simulink library "Common_Library"  (Simulink 8.1)
settings: Solver=ode45  StartTime=0.0  StopTime=10.0  RelTol=1e-3
values from neighbouring files (symbols this model uses):
  address_0x00 = MOVcr    [ROM.m]
  address_0x01 = 10    [ROM.m]
  address_0x02 = REG_A    [ROM.m]
  address_0x03 = MOVcr    [ROM.m]
  address_0x04 = 3    [ROM.m]
  address_0x05 = REG_B    [ROM.m]
  address_0x06 = ADDcr    [ROM.m]
  address_0x07 = 50    [ROM.m]
  address_0x08 = REG_B    [ROM.m]
  address_0x09 = ADDrr    [ROM.m]
  address_0x0A = REG_A    [ROM.m]
  address_0x0B = REG_B    [ROM.m]
  address_0x0C = 0    [ROM.m]
  address_0x0D = 0    [ROM.m]
  address_0x0E = 0    [ROM.m]
  address_0x0F = 177    [ROM.m]
libraries: Common_Library x115, Computer_Library x85, commutil2 x67, simulink_extras x1
(part 3 of 3)

== system Common_Library/Multiplexers/2_to_1_Bit_Multiplexer ==
  Address(1b) : Inport
  Data_In_1(1b) : Inport  Port=2
  Data_In_0(1b) : Inport  Port=3
  Logical Operator12 : Logic  Operator=NOT  Inputs=4  IconShape=distinctive  AllPortsSameDT=off  OutDataTypeStr=boolean
  Logical Operator2 : Logic  IconShape=distinctive  AllPortsSameDT=off  OutDataTypeStr=boolean
  Logical Operator3 : Logic  IconShape=distinctive  AllPortsSameDT=off  OutDataTypeStr=boolean
  Logical Operator8 : Logic  Operator=OR  IconShape=distinctive  OutDataTypeStr=boolean
  Data_Out(1b) : Outport
  wires:
  Logical Operator12/1 -> Logical Operator3/2
  Address(1b)/1 -> Logical Operator2/2, Logical Operator12/1
  Logical Operator8/1 -> Data_Out(1b)/1
  Data_In_1(1b)/1 -> Logical Operator2/1
  Data_In_0(1b)/1 -> Logical Operator3/1
  Logical Operator3/1 -> Logical Operator8/2
  Logical Operator2/1 -> Logical Operator8/1

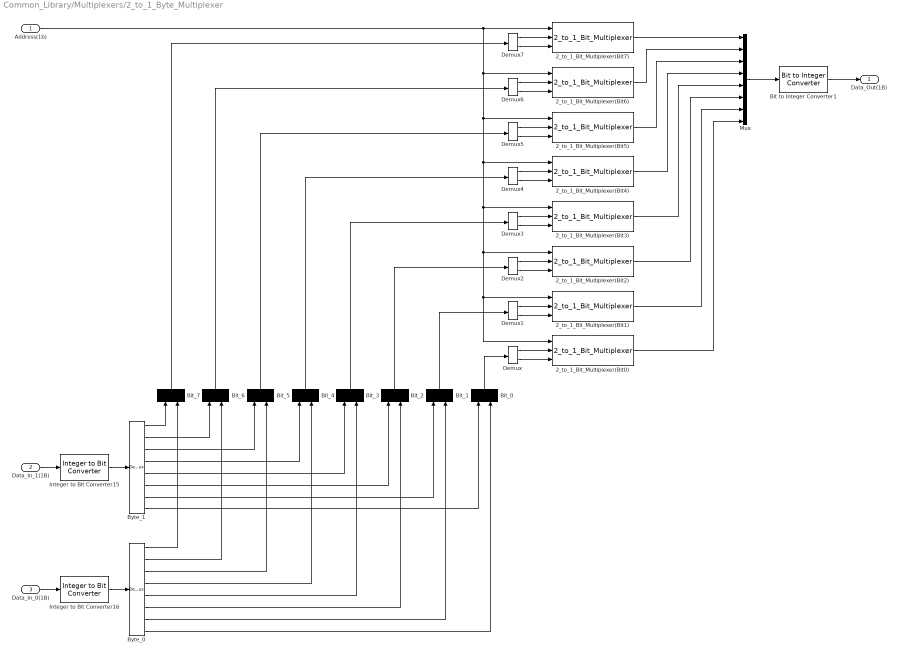
== system Common_Library/Multiplexers/2_to_1_Byte_Multiplexer ==
  Address(1b) : Inport
  Data_In_1(1B) : Inport  Port=2
  Data_In_0(1B) : Inport  Port=3
  2_to_1_Bit_Multiplexer(Bit0) : Common_Library/Multiplexers/2_to_1_Bit_Multiplexer
  2_to_1_Bit_Multiplexer(Bit1) : Common_Library/Multiplexers/2_to_1_Bit_Multiplexer
  2_to_1_Bit_Multiplexer(Bit2) : Common_Library/Multiplexers/2_to_1_Bit_Multiplexer
  2_to_1_Bit_Multiplexer(Bit3) : Common_Library/Multiplexers/2_to_1_Bit_Multiplexer
  2_to_1_Bit_Multiplexer(Bit4) : Common_Library/Multiplexers/2_to_1_Bit_Multiplexer
  2_to_1_Bit_Multiplexer(Bit5) : Common_Library/Multiplexers/2_to_1_Bit_Multiplexer
  2_to_1_Bit_Multiplexer(Bit6) : Common_Library/Multiplexers/2_to_1_Bit_Multiplexer
  2_to_1_Bit_Multiplexer(Bit7) : Common_Library/Multiplexers/2_to_1_Bit_Multiplexer
  Bit to Integer Converter1 : commutil2/Bit to Integer Converter  nbits=8  bitOrder=MSB first  signedOutputValues=Unsigned  outDtype=uint8  outDtypeSigned=Inherit via internal rule
  Bit_{0..7} (8 alike) : Mux  Inputs=2
  Byte_0 : Demux  Outputs=8
  Byte_1 : Demux  Outputs=8
  Demux{,1..7} (8 alike) : Demux  Outputs=2
  Integer to Bit Converter15 : commutil2/Integer to Bit Converter  nbits=8  signedInputValues=Unsigned  bitOrder=MSB first  outDtype=boolean
  Integer to Bit Converter16 : commutil2/Integer to Bit Converter  nbits=8  signedInputValues=Unsigned  bitOrder=MSB first  outDtype=boolean
  Mux : Mux  Inputs=8
  Data_Out(1B) : Outport
  wires:
  Mux/1 -> Bit to Integer Converter1/1
  Bit to Integer Converter1/1 -> Data_Out(1B)/1
  Bit_0/1 -> Demux/1
  Bit_1/1 -> Demux1/1
  Bit_2/1 -> Demux2/1
  Bit_3/1 -> Demux3/1
  Bit_4/1 -> Demux4/1
  Bit_5/1 -> Demux5/1
  Bit_6/1 -> Demux6/1
  Bit_7/1 -> Demux7/1
  Address(1b)/1 -> 2_to_1_Bit_Multiplexer(Bit7)/1, 2_to_1_Bit_Multiplexer(Bit0)/1, 2_to_1_Bit_Multiplexer(Bit1)/1, 2_to_1_Bit_Multiplexer(Bit2)/1, 2_to_1_Bit_Multiplexer(Bit3)/1, 2_to_1_Bit_Multiplexer(Bit4)/1, 2_to_1_Bit_Multiplexer(Bit5)/1, 2_to_1_Bit_Multiplexer(Bit6)/1
  2_to_1_Bit_Multiplexer(Bit4)/1 -> Mux/4
  2_to_1_Bit_Multiplexer(Bit5)/1 -> Mux/3
  2_to_1_Bit_Multiplexer(Bit6)/1 -> Mux/2
  2_to_1_Bit_Multiplexer(Bit7)/1 -> Mux/1
  2_to_1_Bit_Multiplexer(Bit3)/1 -> Mux/5
  2_to_1_Bit_Multiplexer(Bit2)/1 -> Mux/6
  2_to_1_Bit_Multiplexer(Bit1)/1 -> Mux/7
  2_to_1_Bit_Multiplexer(Bit0)/1 -> Mux/8
  Byte_0/8 -> Bit_0/2
  Byte_1/8 -> Bit_0/1
  Byte_0/7 -> Bit_1/2
  Byte_1/7 -> Bit_1/1
  Byte_0/6 -> Bit_2/2
  Byte_1/6 -> Bit_2/1
  Byte_0/5 -> Bit_3/2
  Byte_1/5 -> Bit_3/1
  Byte_0/4 -> Bit_4/2
  Byte_1/4 -> Bit_4/1
  Byte_0/3 -> Bit_5/2
  Byte_1/3 -> Bit_5/1
  Byte_0/2 -> Bit_6/2
  Byte_1/2 -> Bit_6/1
  Byte_0/1 -> Bit_7/2
  Byte_1/1 -> Bit_7/1
  Integer to Bit Converter15/1 -> Byte_1/1
  Data_In_1(1B)/1 -> Integer to Bit Converter15/1
  Integer to Bit Converter16/1 -> Byte_0/1
  Data_In_0(1B)/1 -> Integer to Bit Converter16/1
  Demux/1 -> 2_to_1_Bit_Multiplexer(Bit0)/2
  Demux/2 -> 2_to_1_Bit_Multiplexer(Bit0)/3
  Demux1/1 -> 2_to_1_Bit_Multiplexer(Bit1)/2
  Demux1/2 -> 2_to_1_Bit_Multiplexer(Bit1)/3
  Demux2/1 -> 2_to_1_Bit_Multiplexer(Bit2)/2
  Demux2/2 -> 2_to_1_Bit_Multiplexer(Bit2)/3
  Demux3/2 -> 2_to_1_Bit_Multiplexer(Bit3)/3
  Demux3/1 -> 2_to_1_Bit_Multiplexer(Bit3)/2
  Demux4/2 -> 2_to_1_Bit_Multiplexer(Bit4)/3
  Demux4/1 -> 2_to_1_Bit_Multiplexer(Bit4)/2
  Demux5/1 -> 2_to_1_Bit_Multiplexer(Bit5)/2
  Demux5/2 -> 2_to_1_Bit_Multiplexer(Bit5)/3
  Demux6/1 -> 2_to_1_Bit_Multiplexer(Bit6)/2
  Demux6/2 -> 2_to_1_Bit_Multiplexer(Bit6)/3
  Demux7/2 -> 2_to_1_Bit_Multiplexer(Bit7)/3
  Demux7/1 -> 2_to_1_Bit_Multiplexer(Bit7)/2

== system Common_Library/Multiplexers/4_to_1_Bit_Multiplexer ==
  Address_1(1b) : Inport
  Address_0(1b) : Inport  Port=2
  Data_In_3(1b) : Inport  Port=3
  Data_In_2(1b) : Inport  Port=4
  Data_In_1(1b) : Inport  Port=5
  Data_In_0(1b) : Inport  Port=6
  Logical Operator{,1..3} (4 alike) : Logic  Inputs=3  IconShape=distinctive  AllPortsSameDT=off  OutDataTypeStr=boolean
  Logical Operator11 : Logic  Operator=NOT  Inputs=4  IconShape=distinctive  AllPortsSameDT=off  OutDataTypeStr=boolean
  Logical Operator12 : Logic  Operator=NOT  Inputs=4  IconShape=distinctive  AllPortsSameDT=off  OutDataTypeStr=boolean
  Logical Operator8 : Logic  Operator=OR  Inputs=4  IconShape=distinctive  OutDataTypeStr=boolean
  Data_Out(1b) : Outport
  wires:
  Logical Operator12/1 -> Logical Operator3/2, Logical Operator1/2
  Address_0(1b)/1 -> Logical Operator/2, Logical Operator2/2, Logical Operator12/1
  Logical Operator11/1 -> Logical Operator3/3, Logical Operator2/3
  Address_1(1b)/1 -> Logical Operator/3, Logical Operator1/3, Logical Operator11/1
  Logical Operator8/1 -> Data_Out(1b)/1
  Data_In_3(1b)/1 -> Logical Operator/1
  Data_In_2(1b)/1 -> Logical Operator1/1
  Data_In_1(1b)/1 -> Logical Operator2/1
  Data_In_0(1b)/1 -> Logical Operator3/1
  Logical Operator3/1 -> Logical Operator8/4
  Logical Operator2/1 -> Logical Operator8/3
  Logical Operator1/1 -> Logical Operator8/2
  Logical Operator/1 -> Logical Operator8/1

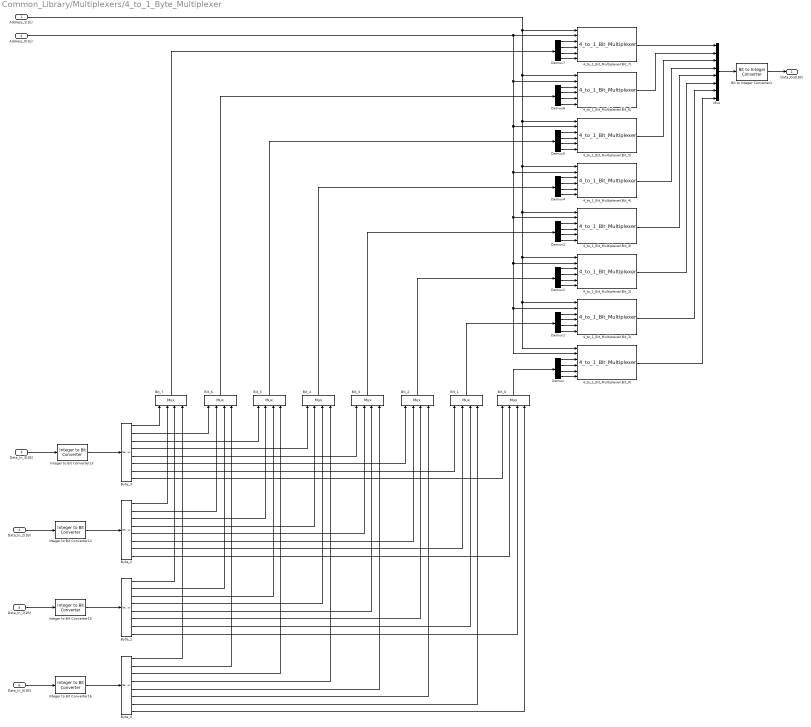
== system Common_Library/Multiplexers/4_to_1_Byte_Multiplexer ==
  Address_1(1b) : Inport
  Address_0(1b) : Inport  Port=2
  Data_In_3(1B) : Inport  Port=3
  Data_In_2(1B) : Inport  Port=4
  Data_In_1(1B) : Inport  Port=5
  Data_In_0(1B) : Inport  Port=6
  4_to_1_Bit_Multiplexer(Bit_0) : Common_Library/Multiplexers/4_to_1_Bit_Multiplexer
  4_to_1_Bit_Multiplexer(Bit_1) : Common_Library/Multiplexers/4_to_1_Bit_Multiplexer
  4_to_1_Bit_Multiplexer(Bit_2) : Common_Library/Multiplexers/4_to_1_Bit_Multiplexer
  4_to_1_Bit_Multiplexer(Bit_3) : Common_Library/Multiplexers/4_to_1_Bit_Multiplexer
  4_to_1_Bit_Multiplexer(Bit_4) : Common_Library/Multiplexers/4_to_1_Bit_Multiplexer
  4_to_1_Bit_Multiplexer(Bit_5) : Common_Library/Multiplexers/4_to_1_Bit_Multiplexer
  4_to_1_Bit_Multiplexer(Bit_6) : Common_Library/Multiplexers/4_to_1_Bit_Multiplexer
  4_to_1_Bit_Multiplexer(Bit_7) : Common_Library/Multiplexers/4_to_1_Bit_Multiplexer
  Bit to Integer Converter1 : commutil2/Bit to Integer Converter  nbits=8  bitOrder=MSB first  signedOutputValues=Unsigned  outDtype=uint8  outDtypeSigned=Inherit via internal rule
  Bit_{0..7} (8 alike) : Mux
  Byte_{0..3} (4 alike) : Demux  Outputs=8
  Demux{,1..7} (8 alike) : Demux
  Integer to Bit Converter{13..16} (4 alike) : commutil2/Integer to Bit Converter  nbits=8  signedInputValues=Unsigned  bitOrder=MSB first  outDtype=boolean
  Mux : Mux  Inputs=8
  Data_Out(1B) : Outport
  wires:
  Mux/1 -> Bit to Integer Converter1/1
  Bit to Integer Converter1/1 -> Data_Out(1B)/1
  Bit_0/1 -> Demux/1
  Bit_1/1 -> Demux1/1
  Bit_2/1 -> Demux2/1
  Bit_3/1 -> Demux3/1
  Bit_4/1 -> Demux4/1
  Bit_5/1 -> Demux5/1
  Bit_6/1 -> Demux6/1
  Bit_7/1 -> Demux7/1
  Address_0(1b)/1 -> 4_to_1_Bit_Multiplexer(Bit_7)/2, 4_to_1_Bit_Multiplexer(Bit_0)/2, 4_to_1_Bit_Multiplexer(Bit_1)/2, 4_to_1_Bit_Multiplexer(Bit_2)/2, 4_to_1_Bit_Multiplexer(Bit_3)/2, 4_to_1_Bit_Multiplexer(Bit_4)/2, 4_to_1_Bit_Multiplexer(Bit_5)/2, 4_to_1_Bit_Multiplexer(Bit_6)/2
  Address_1(1b)/1 -> 4_to_1_Bit_Multiplexer(Bit_7)/1, 4_to_1_Bit_Multiplexer(Bit_0)/1, 4_to_1_Bit_Multiplexer(Bit_1)/1, 4_to_1_Bit_Multiplexer(Bit_2)/1, 4_to_1_Bit_Multiplexer(Bit_3)/1, 4_to_1_Bit_Multiplexer(Bit_4)/1, 4_to_1_Bit_Multiplexer(Bit_5)/1, 4_to_1_Bit_Multiplexer(Bit_6)/1
  4_to_1_Bit_Multiplexer(Bit_4)/1 -> Mux/4
  4_to_1_Bit_Multiplexer(Bit_5)/1 -> Mux/3
  4_to_1_Bit_Multiplexer(Bit_6)/1 -> Mux/2
  4_to_1_Bit_Multiplexer(Bit_7)/1 -> Mux/1
  4_to_1_Bit_Multiplexer(Bit_3)/1 -> Mux/5
  4_to_1_Bit_Multiplexer(Bit_2)/1 -> Mux/6
  4_to_1_Bit_Multiplexer(Bit_1)/1 -> Mux/7
  4_to_1_Bit_Multiplexer(Bit_0)/1 -> Mux/8
  Byte_0/8 -> Bit_0/4
  Byte_1/8 -> Bit_0/3
  Byte_2/8 -> Bit_0/2
  Byte_3/8 -> Bit_0/1
  Byte_0/7 -> Bit_1/4
  Byte_1/7 -> Bit_1/3
  Byte_2/7 -> Bit_1/2
  Byte_3/7 -> Bit_1/1
  Byte_0/6 -> Bit_2/4
  Byte_1/6 -> Bit_2/3
  Byte_2/6 -> Bit_2/2
  Byte_3/6 -> Bit_2/1
  Byte_0/5 -> Bit_3/4
  Byte_1/5 -> Bit_3/3
  Byte_2/5 -> Bit_3/2
  Byte_3/5 -> Bit_3/1
  Byte_0/4 -> Bit_4/4
  Byte_1/4 -> Bit_4/3
  Byte_2/4 -> Bit_4/2
  Byte_3/4 -> Bit_4/1
  Byte_0/3 -> Bit_5/4
  Byte_1/3 -> Bit_5/3
  Byte_2/3 -> Bit_5/2
  Byte_3/3 -> Bit_5/1
  Byte_0/2 -> Bit_6/4
  Byte_1/2 -> Bit_6/3
  Byte_2/2 -> Bit_6/2
  Byte_3/2 -> Bit_6/1
  Byte_0/1 -> Bit_7/4
  Byte_1/1 -> Bit_7/3
  Byte_2/1 -> Bit_7/2
  Byte_3/1 -> Bit_7/1
  Integer to Bit Converter13/1 -> Byte_3/1
  Data_In_3(1B)/1 -> Integer to Bit Converter13/1
  Integer to Bit Converter14/1 -> Byte_2/1
  Data_In_2(1B)/1 -> Integer to Bit Converter14/1
  Integer to Bit Converter15/1 -> Byte_1/1
  Data_In_1(1B)/1 -> Integer to Bit Converter15/1
  Integer to Bit Converter16/1 -> Byte_0/1
  Data_In_0(1B)/1 -> Integer to Bit Converter16/1
  Demux/1 -> 4_to_1_Bit_Multiplexer(Bit_0)/3
  Demux/2 -> 4_to_1_Bit_Multiplexer(Bit_0)/4
  Demux/3 -> 4_to_1_Bit_Multiplexer(Bit_0)/5
  Demux/4 -> 4_to_1_Bit_Multiplexer(Bit_0)/6
  Demux1/1 -> 4_to_1_Bit_Multiplexer(Bit_1)/3
  Demux1/2 -> 4_to_1_Bit_Multiplexer(Bit_1)/4
  Demux1/3 -> 4_to_1_Bit_Multiplexer(Bit_1)/5
  Demux1/4 -> 4_to_1_Bit_Multiplexer(Bit_1)/6
  Demux2/1 -> 4_to_1_Bit_Multiplexer(Bit_2)/3
  Demux2/2 -> 4_to_1_Bit_Multiplexer(Bit_2)/4
  Demux2/3 -> 4_to_1_Bit_Multiplexer(Bit_2)/5
  Demux2/4 -> 4_to_1_Bit_Multiplexer(Bit_2)/6
  Demux3/1 -> 4_to_1_Bit_Multiplexer(Bit_3)/3
  Demux3/2 -> 4_to_1_Bit_Multiplexer(Bit_3)/4
  Demux3/3 -> 4_to_1_Bit_Multiplexer(Bit_3)/5
  Demux3/4 -> 4_to_1_Bit_Multiplexer(Bit_3)/6
  Demux4/1 -> 4_to_1_Bit_Multiplexer(Bit_4)/3
  Demux4/2 -> 4_to_1_Bit_Multiplexer(Bit_4)/4
  Demux4/3 -> 4_to_1_Bit_Multiplexer(Bit_4)/5
  Demux4/4 -> 4_to_1_Bit_Multiplexer(Bit_4)/6
  Demux5/1 -> 4_to_1_Bit_Multiplexer(Bit_5)/3
  Demux5/2 -> 4_to_1_Bit_Multiplexer(Bit_5)/4
  Demux5/3 -> 4_to_1_Bit_Multiplexer(Bit_5)/5
  Demux5/4 -> 4_to_1_Bit_Multiplexer(Bit_5)/6
  Demux6/1 -> 4_to_1_Bit_Multiplexer(Bit_6)/3
  Demux6/2 -> 4_to_1_Bit_Multiplexer(Bit_6)/4
  Demux6/3 -> 4_to_1_Bit_Multiplexer(Bit_6)/5
  Demux6/4 -> 4_to_1_Bit_Multiplexer(Bit_6)/6
  Demux7/1 -> 4_to_1_Bit_Multiplexer(Bit_7)/3
  Demux7/2 -> 4_to_1_Bit_Multiplexer(Bit_7)/4
  Demux7/3 -> 4_to_1_Bit_Multiplexer(Bit_7)/5
  Demux7/4 -> 4_to_1_Bit_Multiplexer(Bit_7)/6

== system Common_Library/Multiplexers/8_to_1_Bit_Multiplexer ==
  Address_2(1b) : Inport
  Address_1(1b) : Inport  Port=2
  Address_0(1b) : Inport  Port=3
  Data_In_7(1b) : Inport  Port=4
  Data_In_6(1b) : Inport  Port=5
  Data_In_5(1b) : Inport  Port=6
  Data_In_4(1b) : Inport  Port=7
  Data_In_3(1b) : Inport  Port=8
  Data_In_2(1b) : Inport  Port=9
  Data_In_1(1b) : Inport  Port=10
  Data_In_0(1b) : Inport  Port=11
  Logical Operator{,1..7} (8 alike) : Logic  Inputs=4  IconShape=distinctive  AllPortsSameDT=off  OutDataTypeStr=boolean
  Logical Operator10 : Logic  Operator=NOT  Inputs=4  IconShape=distinctive  AllPortsSameDT=off  OutDataTypeStr=boolean
  Logical Operator11 : Logic  Operator=NOT  Inputs=4  IconShape=distinctive  AllPortsSameDT=off  OutDataTypeStr=boolean
  Logical Operator12 : Logic  Operator=NOT  Inputs=4  IconShape=distinctive  AllPortsSameDT=off  OutDataTypeStr=boolean
  Logical Operator8 : Logic  Operator=OR  Inputs=8  IconShape=distinctive  OutDataTypeStr=boolean
  Data_Out(1b) : Outport
  wires:
  Logical Operator12/1 -> Logical Operator1/2, Logical Operator3/2, Logical Operator5/2, Logical Operator7/2
  Address_0(1b)/1 -> Logical Operator/2, Logical Operator2/2, Logical Operator4/2, Logical Operator6/2, Logical Operator12/1
  Logical Operator11/1 -> Logical Operator2/4, Logical Operator3/4, Logical Operator6/4, Logical Operator7/4
  Address_1(1b)/1 -> Logical Operator1/4, Logical Operator4/4, Logical Operator5/4, Logical Operator/4, Logical Operator11/1
  Logical Operator10/1 -> Logical Operator4/3, Logical Operator5/3, Logical Operator6/3, Logical Operator7/3
  Address_2(1b)/1 -> Logical Operator3/3, Logical Operator2/3, Logical Operator1/3, Logical Operator/3, Logical Operator10/1
  Logical Operator8/1 -> Data_Out(1b)/1
  Data_In_7(1b)/1 -> Logical Operator/1
  Data_In_6(1b)/1 -> Logical Operator1/1
  Data_In_5(1b)/1 -> Logical Operator2/1
  Data_In_4(1b)/1 -> Logical Operator3/1
  Data_In_3(1b)/1 -> Logical Operator4/1
  Data_In_2(1b)/1 -> Logical Operator5/1
  Data_In_1(1b)/1 -> Logical Operator6/1
  Data_In_0(1b)/1 -> Logical Operator7/1
  Logical Operator7/1 -> Logical Operator8/8
  Logical Operator6/1 -> Logical Operator8/7
  Logical Operator5/1 -> Logical Operator8/6
  Logical Operator4/1 -> Logical Operator8/5
  Logical Operator3/1 -> Logical Operator8/4
  Logical Operator2/1 -> Logical Operator8/3
  Logical Operator1/1 -> Logical Operator8/2
  Logical Operator/1 -> Logical Operator8/1

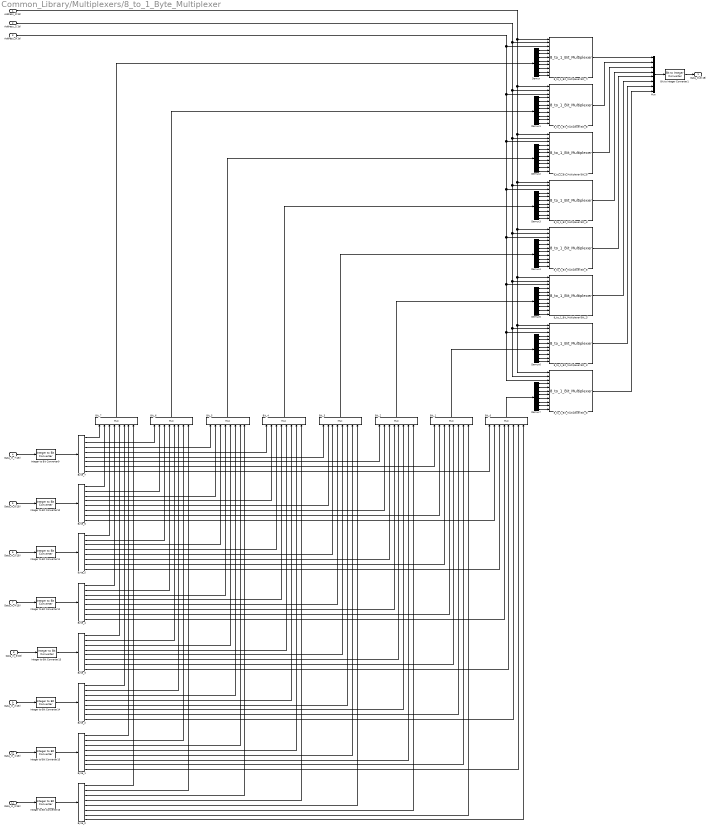
== system Common_Library/Multiplexers/8_to_1_Byte_Multiplexer ==
  Address_2(1b) : Inport
  Address_1(1b) : Inport  Port=2
  Address_0(1b) : Inport  Port=3
  Data_In_7(1B) : Inport  Port=4
  Data_In_6(1B) : Inport  Port=5
  Data_In_5(1B) : Inport  Port=6
  Data_In_4(1B) : Inport  Port=7
  Data_In_3(1B) : Inport  Port=8
  Data_In_2(1B) : Inport  Port=9
  Data_In_1(1B) : Inport  Port=10
  Data_In_0(1B) : Inport  Port=11
  8_to_1_Bit_Multiplexer(Bit_0) : Common_Library/Multiplexers/8_to_1_Bit_Multiplexer
  8_to_1_Bit_Multiplexer(Bit_1) : Common_Library/Multiplexers/8_to_1_Bit_Multiplexer
  8_to_1_Bit_Multiplexer(Bit_2) : Common_Library/Multiplexers/8_to_1_Bit_Multiplexer
  8_to_1_Bit_Multiplexer(Bit_3) : Common_Library/Multiplexers/8_to_1_Bit_Multiplexer
  8_to_1_Bit_Multiplexer(Bit_4) : Common_Library/Multiplexers/8_to_1_Bit_Multiplexer
  8_to_1_Bit_Multiplexer(Bit_5) : Common_Library/Multiplexers/8_to_1_Bit_Multiplexer
  8_to_1_Bit_Multiplexer(Bit_6) : Common_Library/Multiplexers/8_to_1_Bit_Multiplexer
  8_to_1_Bit_Multiplexer(Bit_7) : Common_Library/Multiplexers/8_to_1_Bit_Multiplexer
  Bit to Integer Converter1 : commutil2/Bit to Integer Converter  nbits=8  bitOrder=MSB first  signedOutputValues=Unsigned  outDtype=uint8  outDtypeSigned=Inherit via internal rule
  Bit_{0..7} (8 alike) : Mux  Inputs=8
  Byte_{0..7} (8 alike) : Demux  Outputs=8
  Demux{,1..7} (8 alike) : Demux  Outputs=8
  Integer to Bit Converter{9..16} (8 alike) : commutil2/Integer to Bit Converter  nbits=8  signedInputValues=Unsigned  bitOrder=MSB first  outDtype=boolean
  Mux : Mux  Inputs=8
  Data_Out(1B) : Outport
  wires:
  Mux/1 -> Bit to Integer Converter1/1
  Bit to Integer Converter1/1 -> Data_Out(1B)/1
  Bit_0/1 -> Demux7/1
  Bit_1/1 -> Demux6/1
  Bit_2/1 -> Demux5/1
  Bit_3/1 -> Demux4/1
  Bit_4/1 -> Demux3/1
  Bit_5/1 -> Demux2/1
  Bit_6/1 -> Demux1/1
  Bit_7/1 -> Demux/1
  Byte_7/7 -> Bit_1/1
  Address_0(1b)/1 -> 8_to_1_Bit_Multiplexer(Bit_0)/3, 8_to_1_Bit_Multiplexer(Bit_1)/3, 8_to_1_Bit_Multiplexer(Bit_2)/3, 8_to_1_Bit_Multiplexer(Bit_3)/3, 8_to_1_Bit_Multiplexer(Bit_4)/3, 8_to_1_Bit_Multiplexer(Bit_5)/3, 8_to_1_Bit_Multiplexer(Bit_6)/3, 8_to_1_Bit_Multiplexer(Bit_7)/3
  Address_1(1b)/1 -> 8_to_1_Bit_Multiplexer(Bit_5)/2, 8_to_1_Bit_Multiplexer(Bit_0)/2, 8_to_1_Bit_Multiplexer(Bit_1)/2, 8_to_1_Bit_Multiplexer(Bit_2)/2, 8_to_1_Bit_Multiplexer(Bit_3)/2, 8_to_1_Bit_Multiplexer(Bit_4)/2, 8_to_1_Bit_Multiplexer(Bit_6)/2, 8_to_1_Bit_Multiplexer(Bit_7)/2
  Address_2(1b)/1 -> 8_to_1_Bit_Multiplexer(Bit_0)/1, 8_to_1_Bit_Multiplexer(Bit_1)/1, 8_to_1_Bit_Multiplexer(Bit_2)/1, 8_to_1_Bit_Multiplexer(Bit_3)/1, 8_to_1_Bit_Multiplexer(Bit_4)/1, 8_to_1_Bit_Multiplexer(Bit_5)/1, 8_to_1_Bit_Multiplexer(Bit_6)/1, 8_to_1_Bit_Multiplexer(Bit_7)/1
  8_to_1_Bit_Multiplexer(Bit_4)/1 -> Mux/4
  8_to_1_Bit_Multiplexer(Bit_5)/1 -> Mux/3
  8_to_1_Bit_Multiplexer(Bit_6)/1 -> Mux/2
  8_to_1_Bit_Multiplexer(Bit_7)/1 -> Mux/1
  8_to_1_Bit_Multiplexer(Bit_3)/1 -> Mux/5
  8_to_1_Bit_Multiplexer(Bit_2)/1 -> Mux/6
  8_to_1_Bit_Multiplexer(Bit_1)/1 -> Mux/7
  8_to_1_Bit_Multiplexer(Bit_0)/1 -> Mux/8
  Byte_0/8 -> Bit_0/8
  Byte_1/8 -> Bit_0/7
  Byte_2/8 -> Bit_0/6
  Byte_3/8 -> Bit_0/5
  Byte_4/8 -> Bit_0/4
  Byte_5/8 -> Bit_0/3
  Byte_6/8 -> Bit_0/2
  Byte_7/8 -> Bit_0/1
  Byte_0/7 -> Bit_1/8
  Byte_1/7 -> Bit_1/7
  Byte_2/7 -> Bit_1/6
  Byte_3/7 -> Bit_1/5
  Byte_4/7 -> Bit_1/4
  Byte_5/7 -> Bit_1/3
  Byte_6/7 -> Bit_1/2
  Byte_0/6 -> Bit_2/8
  Byte_1/6 -> Bit_2/7
  Byte_2/6 -> Bit_2/6
  Byte_3/6 -> Bit_2/5
  Byte_4/6 -> Bit_2/4
  Byte_5/6 -> Bit_2/3
  Byte_6/6 -> Bit_2/2
  Byte_7/6 -> Bit_2/1
  Byte_0/5 -> Bit_3/8
  Byte_1/5 -> Bit_3/7
  Byte_2/5 -> Bit_3/6
  Byte_3/5 -> Bit_3/5
  Byte_4/5 -> Bit_3/4
  Byte_5/5 -> Bit_3/3
  Byte_6/5 -> Bit_3/2
  Byte_7/5 -> Bit_3/1
  Byte_0/4 -> Bit_4/8
  Byte_1/4 -> Bit_4/7
  Byte_2/4 -> Bit_4/6
  Byte_3/4 -> Bit_4/5
  Byte_4/4 -> Bit_4/4
  Byte_5/4 -> Bit_4/3
  Byte_6/4 -> Bit_4/2
  Byte_7/4 -> Bit_4/1
  Byte_0/3 -> Bit_5/8
  Byte_1/3 -> Bit_5/7
  Byte_2/3 -> Bit_5/6
  Byte_3/3 -> Bit_5/5
  Byte_4/3 -> Bit_5/4
  Byte_5/3 -> Bit_5/3
  Byte_6/3 -> Bit_5/2
  Byte_7/3 -> Bit_5/1
  Byte_0/2 -> Bit_6/8
  Byte_1/2 -> Bit_6/7
  Byte_2/2 -> Bit_6/6
  Byte_3/2 -> Bit_6/5
  Byte_4/2 -> Bit_6/4
  Byte_5/2 -> Bit_6/3
  Byte_6/2 -> Bit_6/2
  Byte_7/2 -> Bit_6/1
  Byte_0/1 -> Bit_7/8
  Byte_1/1 -> Bit_7/7
  Byte_2/1 -> Bit_7/6
  Byte_3/1 -> Bit_7/5
  Byte_4/1 -> Bit_7/4
  Byte_5/1 -> Bit_7/3
  Byte_6/1 -> Bit_7/2
  Byte_7/1 -> Bit_7/1
  Integer to Bit Converter9/1 -> Byte_7/1
  Data_In_7(1B)/1 -> Integer to Bit Converter9/1
  Integer to Bit Converter10/1 -> Byte_6/1
  Data_In_6(1B)/1 -> Integer to Bit Converter10/1
  Integer to Bit Converter11/1 -> Byte_5/1
  Data_In_5(1B)/1 -> Integer to Bit Converter11/1
  Integer to Bit Converter12/1 -> Byte_4/1
  Data_In_4(1B)/1 -> Integer to Bit Converter12/1
  Integer to Bit Converter13/1 -> Byte_3/1
  Data_In_3(1B)/1 -> Integer to Bit Converter13/1
  Integer to Bit Converter14/1 -> Byte_2/1
  Data_In_2(1B)/1 -> Integer to Bit Converter14/1
  Integer to Bit Converter15/1 -> Byte_1/1
  Data_In_1(1B)/1 -> Integer to Bit Converter15/1
  Integer to Bit Converter16/1 -> Byte_0/1
  Data_In_0(1B)/1 -> Integer to Bit Converter16/1
  Demux/1 -> 8_to_1_Bit_Multiplexer(Bit_7)/4
  Demux/2 -> 8_to_1_Bit_Multiplexer(Bit_7)/5
  Demux/3 -> 8_to_1_Bit_Multiplexer(Bit_7)/6
  Demux/4 -> 8_to_1_Bit_Multiplexer(Bit_7)/7
  Demux/5 -> 8_to_1_Bit_Multiplexer(Bit_7)/8
  Demux/6 -> 8_to_1_Bit_Multiplexer(Bit_7)/9
  Demux/7 -> 8_to_1_Bit_Multiplexer(Bit_7)/10
  Demux/8 -> 8_to_1_Bit_Multiplexer(Bit_7)/11
  Demux1/1 -> 8_to_1_Bit_Multiplexer(Bit_6)/4
  Demux1/2 -> 8_to_1_Bit_Multiplexer(Bit_6)/5
  Demux1/3 -> 8_to_1_Bit_Multiplexer(Bit_6)/6
  Demux1/4 -> 8_to_1_Bit_Multiplexer(Bit_6)/7
  Demux1/5 -> 8_to_1_Bit_Multiplexer(Bit_6)/8
  Demux1/6 -> 8_to_1_Bit_Multiplexer(Bit_6)/9
  Demux1/7 -> 8_to_1_Bit_Multiplexer(Bit_6)/10
  Demux1/8 -> 8_to_1_Bit_Multiplexer(Bit_6)/11
  Demux2/1 -> 8_to_1_Bit_Multiplexer(Bit_5)/4
  Demux2/2 -> 8_to_1_Bit_Multiplexer(Bit_5)/5
  Demux2/3 -> 8_to_1_Bit_Multiplexer(Bit_5)/6
  Demux2/4 -> 8_to_1_Bit_Multiplexer(Bit_5)/7
  Demux2/5 -> 8_to_1_Bit_Multiplexer(Bit_5)/8
  Demux2/6 -> 8_to_1_Bit_Multiplexer(Bit_5)/9
  Demux2/7 -> 8_to_1_Bit_Multiplexer(Bit_5)/10
  Demux2/8 -> 8_to_1_Bit_Multiplexer(Bit_5)/11
  Demux3/1 -> 8_to_1_Bit_Multiplexer(Bit_4)/4
  Demux3/2 -> 8_to_1_Bit_Multiplexer(Bit_4)/5
  Demux3/3 -> 8_to_1_Bit_Multiplexer(Bit_4)/6
  Demux3/4 -> 8_to_1_Bit_Multiplexer(Bit_4)/7
  Demux3/5 -> 8_to_1_Bit_Multiplexer(Bit_4)/8
  Demux3/6 -> 8_to_1_Bit_Multiplexer(Bit_4)/9
  Demux3/7 -> 8_to_1_Bit_Multiplexer(Bit_4)/10
  Demux3/8 -> 8_to_1_Bit_Multiplexer(Bit_4)/11
  Demux4/1 -> 8_to_1_Bit_Multiplexer(Bit_3)/4
  Demux4/2 -> 8_to_1_Bit_Multiplexer(Bit_3)/5
  Demux4/3 -> 8_to_1_Bit_Multiplexer(Bit_3)/6
  Demux4/4 -> 8_to_1_Bit_Multiplexer(Bit_3)/7
  Demux4/5 -> 8_to_1_Bit_Multiplexer(Bit_3)/8
  Demux4/6 -> 8_to_1_Bit_Multiplexer(Bit_3)/9
  Demux4/7 -> 8_to_1_Bit_Multiplexer(Bit_3)/10
  Demux4/8 -> 8_to_1_Bit_Multiplexer(Bit_3)/11
  Demux5/1 -> 8_to_1_Bit_Multiplexer(Bit_2)/4
  Demux5/2 -> 8_to_1_Bit_Multiplexer(Bit_2)/5
  Demux5/3 -> 8_to_1_Bit_Multiplexer(Bit_2)/6
  Demux5/4 -> 8_to_1_Bit_Multiplexer(Bit_2)/7
  Demux5/5 -> 8_to_1_Bit_Multiplexer(Bit_2)/8
  Demux5/6 -> 8_to_1_Bit_Multiplexer(Bit_2)/9
  Demux5/7 -> 8_to_1_Bit_Multiplexer(Bit_2)/10
  Demux5/8 -> 8_to_1_Bit_Multiplexer(Bit_2)/11
  Demux6/1 -> 8_to_1_Bit_Multiplexer(Bit_1)/4
  Demux6/2 -> 8_to_1_Bit_Multiplexer(Bit_1)/5
  Demux6/3 -> 8_to_1_Bit_Multiplexer(Bit_1)/6
  Demux6/4 -> 8_to_1_Bit_Multiplexer(Bit_1)/7
  Demux6/5 -> 8_to_1_Bit_Multiplexer(Bit_1)/8
  Demux6/6 -> 8_to_1_Bit_Multiplexer(Bit_1)/9
  Demux6/7 -> 8_to_1_Bit_Multiplexer(Bit_1)/10
  Demux6/8 -> 8_to_1_Bit_Multiplexer(Bit_1)/11
  Demux7/1 -> 8_to_1_Bit_Multiplexer(Bit_0)/4
  Demux7/2 -> 8_to_1_Bit_Multiplexer(Bit_0)/5
  Demux7/3 -> 8_to_1_Bit_Multiplexer(Bit_0)/6
  Demux7/4 -> 8_to_1_Bit_Multiplexer(Bit_0)/7
  Demux7/5 -> 8_to_1_Bit_Multiplexer(Bit_0)/8
  Demux7/6 -> 8_to_1_Bit_Multiplexer(Bit_0)/9
  Demux7/7 -> 8_to_1_Bit_Multiplexer(Bit_0)/10
  Demux7/8 -> 8_to_1_Bit_Multiplexer(Bit_0)/11

== system Common_Library/Multiplexers/__256_to_1_Bit_Multiplexer__ ==
  Address(8b) : Inport
  Data_In(256b) : Inport  Port=2
  16_to_1_Bit_Multiplexer{0..16} (17 alike) : Computer_Library/Multiplexers/16_to_1_Bit_Multiplexer
  Demux16 : Demux  Outputs=16
  Demux17 : Demux  Outputs=8
  Mux : Mux  Inputs=16
  Data_Out(1b) : Outport
  wires:
  Mux/1 -> 16_to_1_Bit_Multiplexer16/5
  Demux16/1 -> 16_to_1_Bit_Multiplexer0/5
  Demux16/2 -> 16_to_1_Bit_Multiplexer1/5
  Demux16/3 -> 16_to_1_Bit_Multiplexer2/5
  Demux16/4 -> 16_to_1_Bit_Multiplexer3/5
  Demux16/5 -> 16_to_1_Bit_Multiplexer4/5
  Demux16/6 -> 16_to_1_Bit_Multiplexer5/5
  Demux16/16 -> 16_to_1_Bit_Multiplexer15/5
  Demux16/15 -> 16_to_1_Bit_Multiplexer14/5
  Demux16/14 -> 16_to_1_Bit_Multiplexer13/5
  Demux16/13 -> 16_to_1_Bit_Multiplexer12/5
  Demux16/12 -> 16_to_1_Bit_Multiplexer11/5
  Demux16/11 -> 16_to_1_Bit_Multiplexer10/5
  Demux16/10 -> 16_to_1_Bit_Multiplexer9/5
  Demux16/9 -> 16_to_1_Bit_Multiplexer8/5
  Demux16/8 -> 16_to_1_Bit_Multiplexer7/5
  Demux16/7 -> 16_to_1_Bit_Multiplexer6/5
  16_to_1_Bit_Multiplexer0/1 -> Mux/1
  16_to_1_Bit_Multiplexer1/1 -> Mux/2
  16_to_1_Bit_Multiplexer2/1 -> Mux/3
  16_to_1_Bit_Multiplexer3/1 -> Mux/4
  16_to_1_Bit_Multiplexer15/1 -> Mux/16
  16_to_1_Bit_Multiplexer14/1 -> Mux/15
  16_to_1_Bit_Multiplexer13/1 -> Mux/14
  16_to_1_Bit_Multiplexer12/1 -> Mux/13
  16_to_1_Bit_Multiplexer11/1 -> Mux/12
  16_to_1_Bit_Multiplexer10/1 -> Mux/11
  16_to_1_Bit_Multiplexer9/1 -> Mux/10
  16_to_1_Bit_Multiplexer8/1 -> Mux/9
  16_to_1_Bit_Multiplexer7/1 -> Mux/8
  16_to_1_Bit_Multiplexer6/1 -> Mux/7
  16_to_1_Bit_Multiplexer5/1 -> Mux/6
  16_to_1_Bit_Multiplexer4/1 -> Mux/5
  Demux17/5 -> 16_to_1_Bit_Multiplexer0/1, 16_to_1_Bit_Multiplexer1/1, 16_to_1_Bit_Multiplexer2/1, 16_to_1_Bit_Multiplexer3/1, 16_to_1_Bit_Multiplexer4/1, 16_to_1_Bit_Multiplexer5/1, 16_to_1_Bit_Multiplexer6/1, 16_to_1_Bit_Multiplexer7/1, 16_to_1_Bit_Multiplexer8/1, 16_to_1_Bit_Multiplexer9/1, 16_to_1_Bit_Multiplexer10/1, 16_to_1_Bit_Multiplexer11/1, 16_to_1_Bit_Multiplexer12/1, 16_to_1_Bit_Multiplexer13/1, 16_to_1_Bit_Multiplexer14/1, 16_to_1_Bit_Multiplexer15/1
  Demux17/6 -> 16_to_1_Bit_Multiplexer1/2, 16_to_1_Bit_Multiplexer2/2, 16_to_1_Bit_Multiplexer3/2, 16_to_1_Bit_Multiplexer4/2, 16_to_1_Bit_Multiplexer5/2, 16_to_1_Bit_Multiplexer6/2, 16_to_1_Bit_Multiplexer7/2, 16_to_1_Bit_Multiplexer8/2, 16_to_1_Bit_Multiplexer9/2, 16_to_1_Bit_Multiplexer10/2, 16_to_1_Bit_Multiplexer11/2, 16_to_1_Bit_Multiplexer12/2, 16_to_1_Bit_Multiplexer13/2, 16_to_1_Bit_Multiplexer14/2, 16_to_1_Bit_Multiplexer15/2, 16_to_1_Bit_Multiplexer0/2
  Demux17/7 -> 16_to_1_Bit_Multiplexer0/3, 16_to_1_Bit_Multiplexer1/3, 16_to_1_Bit_Multiplexer2/3, 16_to_1_Bit_Multiplexer3/3, 16_to_1_Bit_Multiplexer4/3, 16_to_1_Bit_Multiplexer5/3, 16_to_1_Bit_Multiplexer6/3, 16_to_1_Bit_Multiplexer7/3, 16_to_1_Bit_Multiplexer8/3, 16_to_1_Bit_Multiplexer9/3, 16_to_1_Bit_Multiplexer10/3, 16_to_1_Bit_Multiplexer11/3, 16_to_1_Bit_Multiplexer12/3, 16_to_1_Bit_Multiplexer13/3, 16_to_1_Bit_Multiplexer14/3, 16_to_1_Bit_Multiplexer15/3
  Demux17/8 -> 16_to_1_Bit_Multiplexer0/4, 16_to_1_Bit_Multiplexer1/4, 16_to_1_Bit_Multiplexer2/4, 16_to_1_Bit_Multiplexer3/4, 16_to_1_Bit_Multiplexer4/4, 16_to_1_Bit_Multiplexer5/4, 16_to_1_Bit_Multiplexer6/4, 16_to_1_Bit_Multiplexer7/4, 16_to_1_Bit_Multiplexer8/4, 16_to_1_Bit_Multiplexer9/4, 16_to_1_Bit_Multiplexer10/4, 16_to_1_Bit_Multiplexer11/4, 16_to_1_Bit_Multiplexer12/4, 16_to_1_Bit_Multiplexer13/4, 16_to_1_Bit_Multiplexer14/4, 16_to_1_Bit_Multiplexer15/4
  Demux17/4 -> 16_to_1_Bit_Multiplexer16/4
  Demux17/3 -> 16_to_1_Bit_Multiplexer16/3
  Demux17/2 -> 16_to_1_Bit_Multiplexer16/2
  Demux17/1 -> 16_to_1_Bit_Multiplexer16/1
  Address(8b)/1 -> Demux17/1
  Data_In(256b)/1 -> Demux16/1
  16_to_1_Bit_Multiplexer16/1 -> Data_Out(1b)/1

== system Common_Library/Multiplexers/__256_to_1_Byte_Multiplexer__ ==
  Address(1B) : Inport
  Data_In(256B) : Inport  Port=2
  16_to_1_Byte_Multiplexer{,1..16} (17 alike) : Computer_Library/Multiplexers/16_to_1_Byte_Multiplexer
  Demux16 : Demux  Outputs=16
  Demux17 : Demux  Outputs=8
  Integer to Bit Converter7 : commutil2/Integer to Bit Converter  nbits=8  signedInputValues=Unsigned  bitOrder=MSB first  outDtype=boolean
  Mux : Mux  Inputs=16
  Mux1 : Mux
  Mux2 : Mux
  Data_Out(1B) : Outport
  wires:
  Address(1B)/1 -> Integer to Bit Converter7/1
  Integer to Bit Converter7/1 -> Demux17/1
  Mux2/1 -> 16_to_1_Byte_Multiplexer16/1
  Demux17/4 -> Mux2/4
  Demux17/3 -> Mux2/3
  Demux17/2 -> Mux2/2
  Demux17/1 -> Mux2/1
  Mux1/1 -> 16_to_1_Byte_Multiplexer/1, 16_to_1_Byte_Multiplexer2/1, 16_to_1_Byte_Multiplexer3/1, 16_to_1_Byte_Multiplexer4/1, 16_to_1_Byte_Multiplexer5/1, 16_to_1_Byte_Multiplexer6/1, 16_to_1_Byte_Multiplexer7/1, 16_to_1_Byte_Multiplexer8/1, 16_to_1_Byte_Multiplexer9/1, 16_to_1_Byte_Multiplexer10/1, 16_to_1_Byte_Multiplexer11/1, 16_to_1_Byte_Multiplexer12/1, 16_to_1_Byte_Multiplexer13/1, 16_to_1_Byte_Multiplexer14/1, 16_to_1_Byte_Multiplexer15/1, 16_to_1_Byte_Multiplexer1/1
  Demux17/8 -> Mux1/4
  Demux17/7 -> Mux1/3
  Demux17/6 -> Mux1/2
  Demux17/5 -> Mux1/1
  Demux16/16 -> 16_to_1_Byte_Multiplexer15/2
  Demux16/15 -> 16_to_1_Byte_Multiplexer14/2
  Demux16/14 -> 16_to_1_Byte_Multiplexer13/2
  Demux16/13 -> 16_to_1_Byte_Multiplexer12/2
  Demux16/12 -> 16_to_1_Byte_Multiplexer11/2
  Demux16/11 -> 16_to_1_Byte_Multiplexer10/2
  Demux16/10 -> 16_to_1_Byte_Multiplexer9/2
  Demux16/9 -> 16_to_1_Byte_Multiplexer8/2
  Demux16/8 -> 16_to_1_Byte_Multiplexer7/2
  Demux16/7 -> 16_to_1_Byte_Multiplexer6/2
  Demux16/6 -> 16_to_1_Byte_Multiplexer5/2
  Demux16/5 -> 16_to_1_Byte_Multiplexer4/2
  Demux16/4 -> 16_to_1_Byte_Multiplexer3/2
  Demux16/3 -> 16_to_1_Byte_Multiplexer2/2
  Demux16/2 -> 16_to_1_Byte_Multiplexer1/2
  Demux16/1 -> 16_to_1_Byte_Multiplexer/2
  16_to_1_Byte_Multiplexer16/1 -> Data_Out(1B)/1
  Data_In(256B)/1 -> Demux16/1
  Mux/1 -> 16_to_1_Byte_Multiplexer16/2
  16_to_1_Byte_Multiplexer15/1 -> Mux/16
  16_to_1_Byte_Multiplexer14/1 -> Mux/15
  16_to_1_Byte_Multiplexer13/1 -> Mux/14
  16_to_1_Byte_Multiplexer12/1 -> Mux/13
  16_to_1_Byte_Multiplexer11/1 -> Mux/12
  16_to_1_Byte_Multiplexer10/1 -> Mux/11
  16_to_1_Byte_Multiplexer9/1 -> Mux/10
  16_to_1_Byte_Multiplexer8/1 -> Mux/9
  16_to_1_Byte_Multiplexer7/1 -> Mux/8
  16_to_1_Byte_Multiplexer6/1 -> Mux/7
  16_to_1_Byte_Multiplexer5/1 -> Mux/6
  16_to_1_Byte_Multiplexer4/1 -> Mux/5
  16_to_1_Byte_Multiplexer3/1 -> Mux/4
  16_to_1_Byte_Multiplexer2/1 -> Mux/3
  16_to_1_Byte_Multiplexer1/1 -> Mux/2
  16_to_1_Byte_Multiplexer/1 -> Mux/1

== system Common_Library/Subtractors/1_Bit_Subtractor ==
  Data_In_A(1b) : Inport
  Data_In_B(1b) : Inport  Port=2
  Borrow_In(1b) : Inport  Port=3
  Logical Operator : Logic  IconShape=distinctive  AllPortsSameDT=off  OutDataTypeStr=boolean
  Logical Operator1 : Logic  IconShape=distinctive  AllPortsSameDT=off  OutDataTypeStr=boolean
  Logical Operator10 : Logic  Operator=NOT  Inputs=4  IconShape=distinctive  AllPortsSameDT=off  OutDataTypeStr=boolean
  Logical Operator11 : Logic  Operator=NOT  Inputs=4  IconShape=distinctive  AllPortsSameDT=off  OutDataTypeStr=boolean
  Logical Operator2 : Logic  IconShape=distinctive  AllPortsSameDT=off  OutDataTypeStr=boolean
  Logical Operator{3..6} (4 alike) : Logic  Inputs=3  IconShape=distinctive  AllPortsSameDT=off  OutDataTypeStr=boolean
  Logical Operator7 : Logic  Operator=OR  Inputs=4  IconShape=distinctive  AllPortsSameDT=off  OutDataTypeStr=boolean
  Logical Operator8 : Logic  Operator=OR  Inputs=3  IconShape=distinctive  AllPortsSameDT=off  OutDataTypeStr=boolean
  Logical Operator9 : Logic  Operator=NOT  Inputs=4  IconShape=distinctive  AllPortsSameDT=off  OutDataTypeStr=boolean
  Data_Out(1b) : Outport
  Borrow_Out(1b) : Outport  Port=2
  wires:
  Logical Operator11/1 -> Logical Operator4/3, Logical Operator5/3
  Logical Operator10/1 -> Logical Operator3/2, Logical Operator5/2
  Logical Operator9/1 -> Logical Operator3/1, Logical Operator4/1, Logical Operator/1, Logical Operator1/1
  Data_In_A(1b)/1 -> Logical Operator9/1, Logical Operator5/1, Logical Operator6/1
  Data_In_B(1b)/1 -> Logical Operator10/1, Logical Operator4/2, Logical Operator6/2, Logical Operator/2, Logical Operator2/1
  Borrow_In(1b)/1 -> Logical Operator11/1, Logical Operator3/3, Logical Operator6/3, Logical Operator1/2, Logical Operator2/2
  Logical Operator2/1 -> Logical Operator8/3
  Logical Operator1/1 -> Logical Operator8/2
  Logical Operator/1 -> Logical Operator8/1
  Logical Operator8/1 -> Borrow_Out(1b)/1
  Logical Operator7/1 -> Data_Out(1b)/1
  Logical Operator6/1 -> Logical Operator7/4
  Logical Operator5/1 -> Logical Operator7/3
  Logical Operator4/1 -> Logical Operator7/2
  Logical Operator3/1 -> Logical Operator7/1

== system Common_Library/Subtractors/1_Byte_Subtractor ==
  Data_In_A(1B) : Inport
  Data_In_B(1B) : Inport  Port=2
  1_Bit_Subtractor{,1..7} (8 alike) : Common_Library/Subtractors/1_Bit_Subtractor
  Bit to Integer Converter : commutil2/Bit to Integer Converter  nbits=8  bitOrder=MSB first  signedOutputValues=Unsigned  outDtype=uint8  outDtypeSigned=Inherit via internal rule
  Constant : Constant  Value=0
  Demux : Demux  Outputs=8
  Demux1 : Demux  Outputs=8
  Integer to Bit Converter : commutil2/Integer to Bit Converter  nbits=8  signedInputValues=Unsigned  bitOrder=MSB first  outDtype=uint8
  Integer to Bit Converter1 : commutil2/Integer to Bit Converter  nbits=8  signedInputValues=Unsigned  bitOrder=MSB first  outDtype=uint8
  Mux : Mux  Inputs=8
  Data_Out(1B) : Outport
  Borrow_Out(1b) : Outport  Port=2
  wires:
  Bit to Integer Converter/1 -> Data_Out(1B)/1
  Mux/1 -> Bit to Integer Converter/1
  Integer to Bit Converter1/1 -> Demux1/1
  Data_In_B(1B)/1 -> Integer to Bit Converter1/1
  Integer to Bit Converter/1 -> Demux/1
  Data_In_A(1B)/1 -> Integer to Bit Converter/1
  1_Bit_Subtractor6/2 -> 1_Bit_Subtractor7/3
  1_Bit_Subtractor5/2 -> 1_Bit_Subtractor6/3
  1_Bit_Subtractor4/2 -> 1_Bit_Subtractor5/3
  1_Bit_Subtractor3/2 -> 1_Bit_Subtractor4/3
  1_Bit_Subtractor2/2 -> 1_Bit_Subtractor3/3
  1_Bit_Subtractor1/2 -> 1_Bit_Subtractor2/3
  1_Bit_Subtractor/2 -> 1_Bit_Subtractor1/3
  1_Bit_Subtractor7/2 -> Borrow_Out(1b)/1
  Constant/1 -> 1_Bit_Subtractor/3
  Demux1/8 -> 1_Bit_Subtractor/2
  Demux1/7 -> 1_Bit_Subtractor1/2
  Demux1/6 -> 1_Bit_Subtractor2/2
  Demux1/5 -> 1_Bit_Subtractor3/2
  Demux1/4 -> 1_Bit_Subtractor4/2
  Demux1/3 -> 1_Bit_Subtractor5/2
  Demux1/2 -> 1_Bit_Subtractor6/2
  Demux1/1 -> 1_Bit_Subtractor7/2
  Demux/8 -> 1_Bit_Subtractor/1
  Demux/7 -> 1_Bit_Subtractor1/1
  Demux/6 -> 1_Bit_Subtractor2/1
  Demux/5 -> 1_Bit_Subtractor3/1
  Demux/4 -> 1_Bit_Subtractor4/1
  Demux/3 -> 1_Bit_Subtractor5/1
  Demux/2 -> 1_Bit_Subtractor6/1
  Demux/1 -> 1_Bit_Subtractor7/1
  1_Bit_Subtractor3/1 -> Mux/5
  1_Bit_Subtractor4/1 -> Mux/4
  1_Bit_Subtractor5/1 -> Mux/3
  1_Bit_Subtractor2/1 -> Mux/6
  1_Bit_Subtractor1/1 -> Mux/7
  1_Bit_Subtractor/1 -> Mux/8
  1_Bit_Subtractor6/1 -> Mux/2
  1_Bit_Subtractor7/1 -> Mux/1
